simulink model "A2_compare_c_d"  (Simulink 8.7)
settings: Solver=ode45  StartTime=0.0  StopTime=5  MaxStep=1e-3  RelTol=1e-3
values from neighbouring files (symbols this model uses):
  b_1 = 2.39e6    (= 2390000)    [a1_main.m]    (also in a2_main.m; a3_main.m; a4_main.m)
  c_oil = 36.5e6    (= 36500000)    [a1_main.m]    (also in a2_main.m; a3_main.m; a4_main.m)
  c_p = 75e6    (= 75000000)    [a1_main.m]    (also in a2_main.m; a3_main.m; a4_main.m)
  H = sum_H * lin_sys.b    [a2_main.m]    (also in a3_main.m; a4_main.m)
  lin_sys = linmod('A1_Hydropulszylinder',zeros(3,1),0)    [a1_main.m]    (also in a2_main.m; a3_main.m; a4_main.m)
  m_g = m_k + m_p    (= 268.7)    [a1_main.m]    (also in a2_main.m; a3_main.m; a4_main.m)
  PHI = expm(Ta*lin_sys.a)    [a2_main.m]    (also in a3_main.m; a4_main.m)
  Ta = 15e-3    (= 0.015)    [a1_main.m]    (also in a2_main.m; a3_main.m; a4_main.m)
  u_soll = 1e-4    (= 0.0001)    [a2_main.m]
libraries: simulink x1
settings Model: Creator=jinyao  LastModifiedBy=jinyao
settings DataIOCC: LimitDataPoints=off  SaveFormat=Dataset
settings DebuggingCC: UnderspecifiedInitializationDetection=Simplified  MergeDetectMultiDrivingBlocksExec=error
settings HardwareCC: ProdBitPerPointer=64  ProdLargestAtomicFloat=Float  ProdIntDivRoundTo=Zero  ProdEndianess=LittleEndian  ProdWordSize=64  ProdHWDeviceType=Intel->x86-64 (Windows64)
settings ModelReferenceCC: PropagateSignalLabelsOutOfModel=on
settings ConfigComp: CovModelRefEnable=off

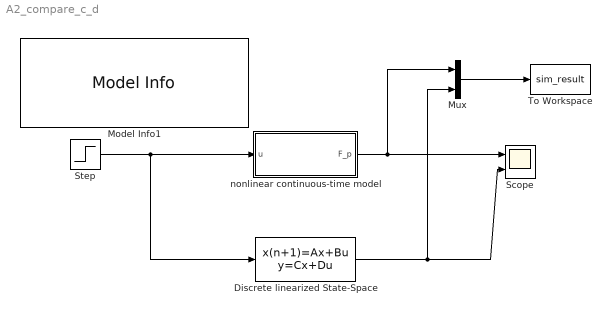
== system A2_compare_c_d ==
  Discrete linearized State-Space : DiscreteStateSpace  A=PHI  B=H  C=lin_sys.c  D=0  SampleTime=Ta
  Model Info1 : simulink/Model-Wide Utilities/Model Info  Frame=on  DisplayStringWithTags=|  HorizontalTextAlignment=Center  LeftAlignmentValue=0.5  SourceBlockDiagram=A2_compare_c_d  TagMaxNumber=20
      | %<ModelName>
      | 
      | MODSIM GRUPPE 11
      | 
      | Cao,Bozhi  Gao,Yue  Jia,Xuehua  Zhu,Jinyao
      | 
      | 14.06.2018
  Mux : Mux  Inputs=2
  Scope : Scope  NumInputPorts=2
  Step : Step  After=u_soll  SampleTime=0
  To Workspace : ToWorkspace  VariableName=sim_result  SaveFormat=Structure With Time  SampleTime=-1
  nonlinear continuous-time model : Subsystem
  wires:
  Discrete linearized State-Space/1 -> Mux/2, Scope/2
  Step/1 -> Discrete linearized State-Space/1, nonlinear continuous-time model/1(u)
  Mux/1 -> To Workspace/1
  nonlinear continuous-time model/1(F_p) -> Mux/1, Scope/1

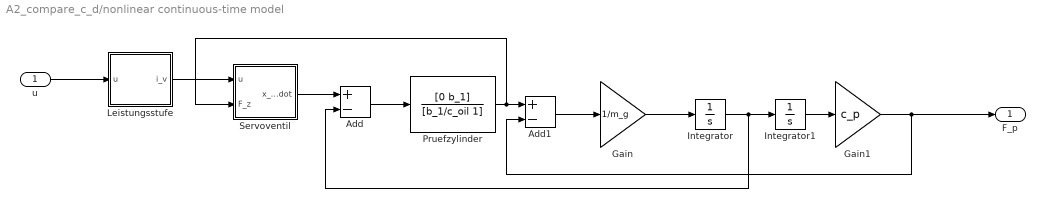
== system A2_compare_c_d/nonlinear continuous-time model ==
  u : Inport
  Add : Sum  Inputs=+-
  Add1 : Sum  Inputs=+-
  Gain : Gain  Gain=1/m_g
  Gain1 : Gain  Gain=c_p
  Integrator : Integrator
  Integrator1 : Integrator
  Leistungsstufe : Subsystem
  Pruefzylinder : TransferFcn  Numerator=[0 b_1]  Denominator=[b_1/c_oil 1]
  Servoventil : Subsystem
  F_p : Outport
  wires:
  Leistungsstufe/1(i_v) -> Servoventil/1(u)
  Servoventil/1(x_oil_dot) -> Add/1
  Add/1 -> Pruefzylinder/1
  Add1/1 -> Gain/1
  Pruefzylinder/1 -> Servoventil/2(F_z), Add1/1
  Gain/1 -> Integrator/1
  Integrator1/1 -> Gain1/1
  Integrator/1 -> Add/2, Integrator1/1
  Gain1/1 -> F_p/1, Add1/2
  u/1 -> Leistungsstufe/1(u)

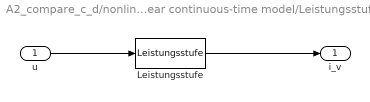
== system A2_compare_c_d/nonlinear continuous-time model/Leistungsstufe ==
  u : Inport
  Leistungsstufe : MATLABFcn  MATLABFcn=Leistungsstufe  OutputDimensions=1  OutputSignalType=real
  i_v : Outport
  wires:
  Leistungsstufe/1 -> i_v/1
  u/1 -> Leistungsstufe/1

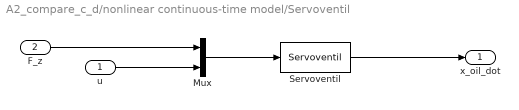
== system A2_compare_c_d/nonlinear continuous-time model/Servoventil ==
  u : Inport
  F_z : Inport  Port=2
  Mux : Mux  Inputs=2
  Servoventil : MATLABFcn  MATLABFcn=Servoventil  OutputDimensions=1  OutputSignalType=real
  x_oil_dot : Outport
  wires:
  Servoventil/1 -> x_oil_dot/1
  u/1 -> Mux/2
  Mux/1 -> Servoventil/1
  F_z/1 -> Mux/1
